simulink model "sub"  (R2018a)
settings: Solver=FixedStepAuto  StartTime=0.0  StopTime=10.0  FixedStep=0.01  RelTol=1e-6
settings Model: Creator=Wang Tianci  LastModifiedBy=Wang Tianci

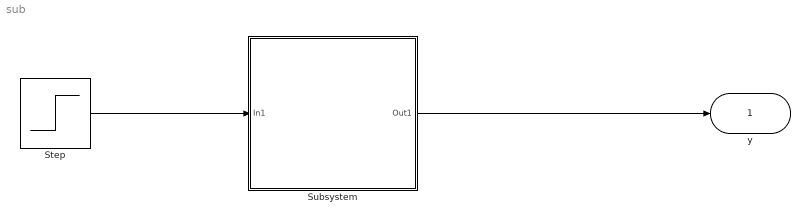
== system sub ==
  Step : Step  SampleTime=0
  Subsystem : Subsystem  mask{a=6}
  "y " : Outport
  wires:
  Step/1 -> Subsystem/1(In1)
  Subsystem/1(Out1) -> "y "/1

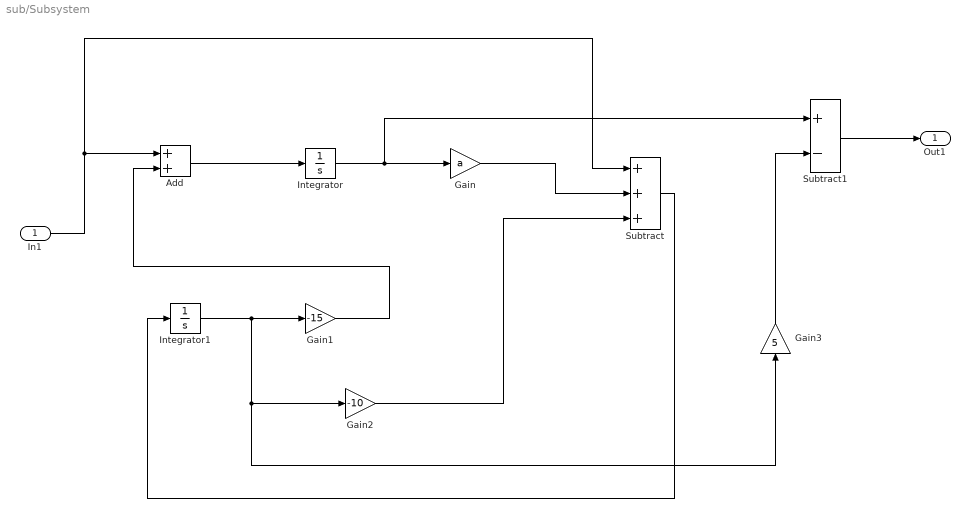
== system sub/Subsystem ==
  In1 : Inport
  Add : Sum
  Gain : Gain  Gain=a
  Gain1 : Gain  Gain=-15
  Gain2 : Gain  Gain=-10
  Gain3 : Gain  Gain=5
  Integrator : Integrator  InitialCondition=1.0
  Integrator1 : Integrator
  Subtract : Sum  Inputs=+++
  Subtract1 : Sum  Inputs=+-
  Out1 : Outport
  wires:
  Add/1 -> Integrator/1
  Integrator1/1 -> Gain1/1, Gain2/1, Gain3/1
  Gain1/1 -> Add/2
  Integrator/1 -> Subtract1/1, Gain/1
  Subtract1/1 -> Out1/1
  Subtract/1 -> Integrator1/1
  Gain2/1 -> Subtract/3
  Gain3/1 -> Subtract1/2
  Gain/1 -> Subtract/2
  In1/1 -> Add/1, Subtract/1
